simulink model "SimulinkFullblock"  (R2019b)
(part 5 of 5)

                                                                                                                                                                                                                                                                                                                                                                                                                                                                                                                                                                                                                                                                                                                                                                                                                                                                                                                                                                                                                                                                                                                                                                                                                                                                                                                                                                                                                                                                                                                                                                                                                                                                                                                                                                                                                                                      0,                                                                                                                                                                                                                                                                                                                                                                                                                                                                                                                                                                                                                                                                                                                                                                                                                                                                                                                                                                                                                                                                                                                                                                                                                                                                                                                                                                                                                                                                                                                                                                                                                                                                                                                                                                                                                                                                                                                                                                                                                                                                                                                                                                                                                                                                                                                                                                                                                                                                                                                                                                                                                                                                                                                                                                                                                                                                                                                                                                                                                                                                                                                                                                                                                                                                                                                                                                                                                                                                                                                                                                                                                                                                                                                                                                                                                                                                                                                                                                                                                                                                                                                                                                                                                                                                                                                                                                                                                                                                                                                                                                                                                                                                                                                                                                                                                                                                               -0.0175*sin(0.0175*q1 - 1.5708)*q1d,                                                                                                                                                         0,                                                                                                                                                                                                                                                                                                                                                                                                                                                                                                                                                                                                                                                                                                                                                                                                                                                                                                                                                                                                                                                                                                                                                                                                                                                                                                                                                                                                                                                                                                                                                                                                                                                                                                                                                                                                                                                                                                                                                                                                                                                                                                                                                                                                                                                                                                                                                                                                                                                                                                                                                                                                                                                                                                                                                                                                                                                                                                                                                                                                                                                                                                                                                                                                                                                                                                                                                                                                                                                                                                                                                                                                                                                                                                                                                                                                                                                                                                                                                                                                                                                                                                                                                                                                                                                                                                                                                                                                                                                                                                                                                                                                                                                                                                                                                                                                                                                                                                                                                                                                                                                                                                                                                                                                                                                                                                                                                                                                                                                                                                                                                                                                                                                                                                                                                                                                                                                                                                                                                                                                                                                                                                                                                                                                                                                                                                                                                                                                                                                                                                                                                                                                                                                                                                                                                                                                                                                                                                                                                                                                                                                                                                                                                                                                 0.0175*cos(0.0175*q1 - 1.5708)*sin(0.0175*q2 - 1.5708)*q1d + 0.0175*cos(0.0175*q2 - 1.5708)*sin(0.0175*q1 - 1.5708)*q2d,                                                                                                                                                                                                                                                                                                                                                                                                                                                                                                                                                                                                                                                                                                                                                                                                                                                                                                                                                                                                                                                                                                                                                                                                                                                                                                                                                                                                                                                                                                                                                                                                                                                                                                                                                                                                                                                                                                                                                                                                                                                                                                                                                                                                                                                                                                                                                                                                                                                                                                                                                                                                                                                                                                                                                                                                                                                                                                                                                                                                                                                                                                                                                                                                                                                                                                                                                                                                                                                                                                                                                                                                                                                                                                                                                                                                                                                                                                                                                                                                                                                                                                                                                                                                                                                                                                                                                                                                                                                                                                                                                                                                                                                                                                                                                                                                                                                                                                                                                                                                                                                                                                                                                                                                                                                                                                                                                                                                                                                                                                                                                                                                                                                                                                                                                                                                                                                                                                                                                                                                                                                                                                                                                                                                                                                                                                                                                                                                                                                                                                                                                                                                                                                                                                                                                                                                                                                                                                                                                                                                                                                                                                                                                                                                                                                                                      0.0175*cos(0.0175*q4 + 1.5708)*sin(0.0175*q1 - 1.5708)*q1d + 0.0175*cos(0.0175*q1 - 1.5708)*sin(0.0175*q4 + 1.5708)*q4d + 0.0175*cos(0.0175*q1 - 1.5708)*cos(0.0175*q2 - 1.5708)*sin(0.0175*q4 + 1.5708)*q1d + 0.0175*cos(0.0175*q2 - 1.5708)*cos(0.0175*q4 + 1.5708)*sin(0.0175*q1 - 1.5708)*q4d - 0.0175*sin(0.0175*q1 - 1.5708)*sin(0.0175*q2 - 1.5708)*sin(0.0175*q4 + 1.5708)*q2d,                                                                                                                                                                                                                                                                                                                                                                                                                                                                                                                                                                                                                                                                                                                                                                                                                                                                                                                                                                                                                                                                                                                                                                                                                                                                                                                                                                                                                                                                                                                                                                                                                                                                                                                                                                                                                                                                                                                                                                                                                                                                                                                                                                                                                                                                                                                                                                                                                                                                                                                                                                                                                                                                                                                                                                                                                                                                                                                                                                                                                                                                                                                                                                                                                                                                                                                                                                                                                                                                                                                                                                                                                                                                                                                                                                                                                                                                                                                                                                                                                                                                                                                                                                                                                                                                                                                                                                                                                                                                                                                                                                                                                                                                                                                                                                                                                                                                                                                                                                                                                                                                                                                                                                                                                                                                                                                                                                                                                                                                                                                                                                                                                                                                                                                                                                                                                                                                                                                                                                                                                                                                                                                                                                                                                                                                                                                                                                                                                                                                                                                                                                                                                                                                                                                                                                                                                                                                                                                                                                                                                                                                                                                                                                                                                                                                                                                                                                                                                                                                                                                                                                                                                                                                                                                                                                                                                                                                                                                                                                                                                                                                                                                                                                                                                                                                                                                                                                            0.0175*cos(0.0175*q5 + 1.5708)*q5d*(cos(0.0175*q1 - 1.5708)*sin(0.0175*q4 + 1.5708) + cos(0.0175*q2 - 1.5708)*cos(0.0175*q4 + 1.5708)*sin(0.0175*q1 - 1.5708)) - sin(0.0175*q5 + 1.5708)*(0.0175*sin(0.0175*q1 - 1.5708)*sin(0.0175*q4 + 1.5708)*q1d - 0.0175*cos(0.0175*q1 - 1.5708)*cos(0.0175*q4 + 1.5708)*q4d - 0.0175*cos(0.0175*q1 - 1.5708)*cos(0.0175*q2 - 1.5708)*cos(0.0175*q4 + 1.5708)*q1d + 0.0175*cos(0.0175*q4 + 1.5708)*sin(0.0175*q1 - 1.5708)*sin(0.0175*q2 - 1.5708)*q2d + 0.0175*cos(0.0175*q2 - 1.5708)*sin(0.0175*q1 - 1.5708)*sin(0.0175*q4 + 1.5708)*q4d) - 0.0175*cos(0.0175*q1 - 1.5708)*cos(0.0175*q5 + 1.5708)*sin(0.0175*q2 - 1.5708)*q1d - 0.0175*cos(0.0175*q2 - 1.5708)*cos(0.0175*q5 + 1.5708)*sin(0.0175*q1 - 1.5708)*q2d + 0.0175*sin(0.0175*q1 - 1.5708)*sin(0.0175*q2 - 1.5708)*sin(0.0175*q5 + 1.5708)*q5d;
                                                                                                                                                                                                                                                                                                                                                                                                                                                                                                                                                                                                                                                                                                                                                                                                                                                                                                                                                                                                                                                                                                                                                                                                                                                                                                                                                                                                                                                                                                                                                                                                                                                                                                                                                                                                                                                      0,                                                                                                                                                                                                                                                                                                                                                                                                                                                                                                                                                                                                                                                                                                                                                                                                                                                                                                                                                                                                                                                                                                                                                                                                                                                                                                                                                                                                                                                                                                                                                                                                                                                                                                                                                                                                                                                                                                                                                                                                                                                                                                                                                                                                                                                                                                                                                                                                                                                                                                                                                                                                                                                                                                                                                                                                                                                                                                                                                                                                                                                                                                                                                                                                                                                                                                                                                                                                                                                                                                                                                                                                                                                                                                                                                                                                                                                                                                                                                                                                                                                                                                                                                                                                                                                                                                                                                                                                                                                                                                                                                                                                                                                                                                                                                                                                                                                                                                                               0,                                                                                                                                                         0,                                                                                                                                                                                                                                                                                                                                                                                                                                                                                                                                                                                                                                                                                                                                                                                                                                                                                                                                                                                                                                                                                                                                                                                                                                                                                                                                                                                                                                                                                                                                                                                                                                                                                                                                                                                                                                                                                                                                                                                                                                                                                                                                                                                                                                                                                                                                                                                                                                                                                                                                                                                                                                                                                                                                                                                                                                                                                                                                                                                                                                                                                                                                                                                                                                                                                                                                                                                                                                                                                                                                                                                                                                                                                                                                                                                                                                                                                                                                                                                                                                                                                                                                                                                                                                                                                                                                                                                                                                                                                                                                                                                                                                                                                                                                                                                                                                                                                                                                                                                                                                                                                                                                                                                                                                                                                                                                                                                                                                                                                                                                                                                                                                                                                                                                                                                                                                                                                                                                                                                                                                                                                                                                                                                                                                                                                                                                                                                                                                                                                                                                                                                                                                                                                                                                                                                                                                                                                                                                                                                                                                                                                                                                                                                                                                                                                                         -0.0175*sin(0.0175*q2 - 1.5708)*q2d,                                                                                                                                                                                                                                                                                                                                                                                                                                                                                                                                                                                                                                                                                                                                                                                                                                                                                                                                                                                                                                                                                                                                                                                                                                                                                                                                                                                                                                                                                                                                                                                                                                                                                                                                                                                                                                                                                                                                                                                                                                                                                                                                                                                                                                                                                                                                                                                                                                                                                                                                                                                                                                                                                                                                                                                                                                                                                                                                                                                                                                                                                                                                                                                                                                                                                                                                                                                                                                                                                                                                                                                                                                                                                                                                                                                                                                                                                                                                                                                                                                                                                                                                                                                                                                                                                                                                                                                                                                                                                                                                                                                                                                                                                                                                                                                                                                                                                                                                                                                                                                                                                                                                                                                                                                                                                                                                                                                                                                                                                                                                                                                                                                                                                                                                                                                                                                                                                                                                                                                                                                                                                                                                                                                                                                                                                                                                                                                                                                                                                                                                                                                                                                                                                                                                                                                                                                                                                                                                                                                                                                                                                                                                                                                                                                                                                                                                                                                                                                                                                                                                                                                                               - 0.0175*cos(0.0175*q2 - 1.5708)*sin(0.0175*q4 + 1.5708)*q2d - 0.0175*cos(0.0175*q4 + 1.5708)*sin(0.0175*q2 - 1.5708)*q4d,                                                                                                                                                                                                                                                                                                                                                                                                                                                                                                                                                                                                                                                                                                                                                                                                                                                                                                                                                                                                                                                                                                                                                                                                                                                                                                                                                                                                                                                                                                                                                                                                                                                                                                                                                                                                                                                                                                                                                                                                                                                                                                                                                                                                                                                                                                                                                                                                                                                                                                                                                                                                                                                                                                                                                                                                                                                                                                                                                                                                                                                                                                                                                                                                                                                                                                                                                                                                                                                                                                                                                                                                                                                                                                                                                                                                                                                                                                                                                                                                                                                                                                                                                                                                                                                                                                                                                                                                                                                                                                                                                                                                                                                                                                                                                                                                                                                                                                                                                                                                                                                                                                                                                                                                                                                                                                                                                                                                                                                                                                                                                                                                                                                                                                                                                                                                                                                                                                                                                                                                                                                                                                                                                                                                                                                                                                                                                                                                                                                                                                                                                                                                                                                                                                                                                                                                                                                                                                                                                                                                                                                                                                                                                                                                                                                                                                                                                                                                                                                                                                                                                                                                                                                                                                                                                                                                                                                                                                                                                                                                                                                                                                                                                                                                                                                                                                                                                                                                                                                                                                                                                                                                                                                                                                                                                                                                                                                                                                                                  0.0175*cos(0.0175*q5 + 1.5708)*sin(0.0175*q2 - 1.5708)*q2d + 0.0175*cos(0.0175*q2 - 1.5708)*sin(0.0175*q5 + 1.5708)*q5d - 0.0175*cos(0.0175*q2 - 1.5708)*cos(0.0175*q4 + 1.5708)*sin(0.0175*q5 + 1.5708)*q2d - 0.0175*cos(0.0175*q4 + 1.5708)*cos(0.0175*q5 + 1.5708)*sin(0.0175*q2 - 1.5708)*q5d + 0.0175*sin(0.0175*q2 - 1.5708)*sin(0.0175*q4 + 1.5708)*sin(0.0175*q5 + 1.5708)*q4d];
                                                                                                                                                                                                                                                                                                                                                                                                                                                                                                                                                                                                                                                                                                                                                                                                                                                                                                                                                                                                                                                                                                                                                                                                                                                                                                                                                                                                                                                                                                                                                                                                                                                                                                                                                                                                                                                  
                                                                                                                                                                                                                                                                                                                                                                                                                                                                                                                                                                                                                                                                                                                                                                                                                                                                                                                                                                                                                                                                                                                                                                                                                                                                                                                                                                                                                                                                                                                                                                                                                                                                                                                             

J= [ - conj(L4)*(sin(0.0175*conj(q5) + 1.5708)*(cos(0.0175*conj(q1) - 1.5708)*sin(0.0175*conj(q4) + 1.5708) + cos(0.0175*conj(q2) - 1.5708)*cos(0.0175*conj(q4) + 1.5708)*sin(0.0175*conj(q1) - 1.5708)) - cos(0.0175*conj(q5) + 1.5708)*sin(0.0175*conj(q1) - 1.5708)*sin(0.0175*conj(q2) - 1.5708)) - sin(0.0175*conj(q1) - 1.5708)*sin(0.0175*conj(q2) - 1.5708)*(conj(q3) + conj(L2)) - sin(0.0175*conj(q1) - 1.5708)*sin(0.0175*conj(q2) - 1.5708)*conj(L3),                                                                                                                                                                                                                                                                                                                                                                                                                                                                                                                                                                                                                                                                                                                                                      cos(0.0175*conj(q1) - 1.5708)*(cos(0.0175*conj(q2) - 1.5708)*conj(L3) - conj(L4)*(cos(0.0175*conj(q2) - 1.5708)*cos(0.0175*conj(q5) + 1.5708) + cos(0.0175*conj(q4) + 1.5708)*sin(0.0175*conj(q2) - 1.5708)*sin(0.0175*conj(q5) + 1.5708)) + cos(0.0175*conj(q2) - 1.5708)*(conj(q3) + conj(L2))), cos(0.0175*q1 - 1.5708)*sin(0.0175*q2 - 1.5708),                                                                                                                                                                                                                                                                             sin(0.0175*conj(q1) - 1.5708)*sin(0.0175*conj(q2) - 1.5708)*(cos(0.0175*conj(q2) - 1.5708)*conj(L3) - conj(L4)*(cos(0.0175*conj(q2) - 1.5708)*cos(0.0175*conj(q5) + 1.5708) + cos(0.0175*conj(q4) + 1.5708)*sin(0.0175*conj(q2) - 1.5708)*sin(0.0175*conj(q5) + 1.5708)) + cos(0.0175*conj(q2) - 1.5708)*(conj(q3) + conj(L2)) - cos(0.0175*conj(q2) - 1.5708)*(conj(q3) + conj(L2))) - cos(0.0175*conj(q2) - 1.5708)*(conj(L4)*(sin(0.0175*conj(q5) + 1.5708)*(cos(0.0175*conj(q1) - 1.5708)*sin(0.0175*conj(q4) + 1.5708) + cos(0.0175*conj(q2) - 1.5708)*cos(0.0175*conj(q4) + 1.5708)*sin(0.0175*conj(q1) - 1.5708)) - cos(0.0175*conj(q5) + 1.5708)*sin(0.0175*conj(q1) - 1.5708)*sin(0.0175*conj(q2) - 1.5708)) + sin(0.0175*conj(q1) - 1.5708)*sin(0.0175*conj(q2) - 1.5708)*(conj(q3) + conj(L2)) - sin(0.0175*conj(q1) - 1.5708)*sin(0.0175*conj(q2) - 1.5708)*(conj(q3) + conj(L2)) + sin(0.0175*conj(q1) - 1.5708)*sin(0.0175*conj(q2) - 1.5708)*conj(L3)),                                                                                                                                                                                                                                                                                                                                                                                    (cos(0.0175*conj(q1) - 1.5708)*cos(0.0175*conj(q4) + 1.5708) - cos(0.0175*conj(q2) - 1.5708)*sin(0.0175*conj(q1) - 1.5708)*sin(0.0175*conj(q4) + 1.5708))*(cos(0.0175*conj(q2) - 1.5708)*conj(L3) - cos(0.0175*conj(q2) - 1.5708)*conj(L3) + conj(L4)*(cos(0.0175*conj(q2) - 1.5708)*cos(0.0175*conj(q5) + 1.5708) + cos(0.0175*conj(q4) + 1.5708)*sin(0.0175*conj(q2) - 1.5708)*sin(0.0175*conj(q5) + 1.5708)) - cos(0.0175*conj(q2) - 1.5708)*(conj(q3) + conj(L2)) + cos(0.0175*conj(q2) - 1.5708)*(conj(q3) + conj(L2))) + sin(0.0175*conj(q2) - 1.5708)*sin(0.0175*conj(q4) + 1.5708)*(conj(L4)*(sin(0.0175*conj(q5) + 1.5708)*(cos(0.0175*conj(q1) - 1.5708)*sin(0.0175*conj(q4) + 1.5708) + cos(0.0175*conj(q2) - 1.5708)*cos(0.0175*conj(q4) + 1.5708)*sin(0.0175*conj(q1) - 1.5708)) - cos(0.0175*conj(q5) + 1.5708)*sin(0.0175*conj(q1) - 1.5708)*sin(0.0175*conj(q2) - 1.5708)) + sin(0.0175*conj(q1) - 1.5708)*sin(0.0175*conj(q2) - 1.5708)*(conj(q3) + conj(L2)) - sin(0.0175*conj(q1) - 1.5708)*sin(0.0175*conj(q2) - 1.5708)*(conj(q3) + conj(L2)) + sin(0.0175*conj(q1) - 1.5708)*sin(0.0175*conj(q2) - 1.5708)*conj(L3) - sin(0.0175*conj(q1) - 1.5708)*sin(0.0175*conj(q2) - 1.5708)*conj(L3)),                                                                                                                                                                                                                                                                                                                                                                                                                     (cos(0.0175*conj(q2) - 1.5708)*cos(0.0175*conj(q5) + 1.5708) + cos(0.0175*conj(q4) + 1.5708)*sin(0.0175*conj(q2) - 1.5708)*sin(0.0175*conj(q5) + 1.5708))*(conj(L4)*(sin(0.0175*conj(q5) + 1.5708)*(cos(0.0175*conj(q1) - 1.5708)*sin(0.0175*conj(q4) + 1.5708) + cos(0.0175*conj(q2) - 1.5708)*cos(0.0175*conj(q4) + 1.5708)*sin(0.0175*conj(q1) - 1.5708)) - cos(0.0175*conj(q5) + 1.5708)*sin(0.0175*conj(q1) - 1.5708)*sin(0.0175*conj(q2) - 1.5708)) + sin(0.0175*conj(q1) - 1.5708)*sin(0.0175*conj(q2) - 1.5708)*(conj(q3) + conj(L2)) - sin(0.0175*conj(q1) - 1.5708)*sin(0.0175*conj(q2) - 1.5708)*(conj(q3) + conj(L2)) + sin(0.0175*conj(q1) - 1.5708)*sin(0.0175*conj(q2) - 1.5708)*conj(L3) - sin(0.0175*conj(q1) - 1.5708)*sin(0.0175*conj(q2) - 1.5708)*conj(L3)) - (sin(0.0175*conj(q5) + 1.5708)*(cos(0.0175*conj(q1) - 1.5708)*sin(0.0175*conj(q4) + 1.5708) + cos(0.0175*conj(q2) - 1.5708)*cos(0.0175*conj(q4) + 1.5708)*sin(0.0175*conj(q1) - 1.5708)) - cos(0.0175*conj(q5) + 1.5708)*sin(0.0175*conj(q1) - 1.5708)*sin(0.0175*conj(q2) - 1.5708))*(cos(0.0175*conj(q2) - 1.5708)*conj(L3) - cos(0.0175*conj(q2) - 1.5708)*conj(L3) + conj(L4)*(cos(0.0175*conj(q2) - 1.5708)*cos(0.0175*conj(q5) + 1.5708) + cos(0.0175*conj(q4) + 1.5708)*sin(0.0175*conj(q2) - 1.5708)*sin(0.0175*conj(q5) + 1.5708)) - cos(0.0175*conj(q2) - 1.5708)*(conj(q3) + conj(L2)) + cos(0.0175*conj(q2) - 1.5708)*(conj(q3) + conj(L2)));
   cos(0.0175*conj(q1) - 1.5708)*sin(0.0175*conj(q2) - 1.5708)*conj(L3) - conj(L4)*(sin(0.0175*conj(q5) + 1.5708)*(sin(0.0175*conj(q1) - 1.5708)*sin(0.0175*conj(q4) + 1.5708) - cos(0.0175*conj(q1) - 1.5708)*cos(0.0175*conj(q2) - 1.5708)*cos(0.0175*conj(q4) + 1.5708)) + cos(0.0175*conj(q1) - 1.5708)*cos(0.0175*conj(q5) + 1.5708)*sin(0.0175*conj(q2) - 1.5708)) + cos(0.0175*conj(q1) - 1.5708)*sin(0.0175*conj(q2) - 1.5708)*(conj(q3) + conj(L2)),                                                                                                                                                                                                                                                                                                                                                                                                                                                                                                                                                                                                                                                                                                                                                      sin(0.0175*conj(q1) - 1.5708)*(cos(0.0175*conj(q2) - 1.5708)*conj(L3) - conj(L4)*(cos(0.0175*conj(q2) - 1.5708)*cos(0.0175*conj(q5) + 1.5708) + cos(0.0175*conj(q4) + 1.5708)*sin(0.0175*conj(q2) - 1.5708)*sin(0.0175*conj(q5) + 1.5708)) + cos(0.0175*conj(q2) - 1.5708)*(conj(q3) + conj(L2))), sin(0.0175*q1 - 1.5708)*sin(0.0175*q2 - 1.5708),                                                                                                                                                                                                                                                                           - cos(0.0175*conj(q2) - 1.5708)*(conj(L4)*(sin(0.0175*conj(q5) + 1.5708)*(sin(0.0175*conj(q1) - 1.5708)*sin(0.0175*conj(q4) + 1.5708) - cos(0.0175*conj(q1) - 1.5708)*cos(0.0175*conj(q2) - 1.5708)*cos(0.0175*conj(q4) + 1.5708)) + cos(0.0175*conj(q1) - 1.5708)*cos(0.0175*conj(q5) + 1.5708)*sin(0.0175*conj(q2) - 1.5708)) - cos(0.0175*conj(q1) - 1.5708)*sin(0.0175*conj(q2) - 1.5708)*conj(L3) - cos(0.0175*conj(q1) - 1.5708)*sin(0.0175*conj(q2) - 1.5708)*(conj(q3) + conj(L2)) + cos(0.0175*conj(q1) - 1.5708)*sin(0.0175*conj(q2) - 1.5708)*(conj(q3) + conj(L2))) - cos(0.0175*conj(q1) - 1.5708)*sin(0.0175*conj(q2) - 1.5708)*(cos(0.0175*conj(q2) - 1.5708)*conj(L3) - conj(L4)*(cos(0.0175*conj(q2) - 1.5708)*cos(0.0175*conj(q5) + 1.5708) + cos(0.0175*conj(q4) + 1.5708)*sin(0.0175*conj(q2) - 1.5708)*sin(0.0175*conj(q5) + 1.5708)) + cos(0.0175*conj(q2) - 1.5708)*(conj(q3) + conj(L2)) - cos(0.0175*conj(q2) - 1.5708)*(conj(q3) + conj(L2))),                                                                                                                                                                                                                                                                                                                                                                                    (cos(0.0175*conj(q4) + 1.5708)*sin(0.0175*conj(q1) - 1.5708) + cos(0.0175*conj(q1) - 1.5708)*cos(0.0175*conj(q2) - 1.5708)*sin(0.0175*conj(q4) + 1.5708))*(cos(0.0175*conj(q2) - 1.5708)*conj(L3) - cos(0.0175*conj(q2) - 1.5708)*conj(L3) + conj(L4)*(cos(0.0175*conj(q2) - 1.5708)*cos(0.0175*conj(q5) + 1.5708) + cos(0.0175*conj(q4) + 1.5708)*sin(0.0175*conj(q2) - 1.5708)*sin(0.0175*conj(q5) + 1.5708)) - cos(0.0175*conj(q2) - 1.5708)*(conj(q3) + conj(L2)) + cos(0.0175*conj(q2) - 1.5708)*(conj(q3) + conj(L2))) + sin(0.0175*conj(q2) - 1.5708)*sin(0.0175*conj(q4) + 1.5708)*(conj(L4)*(sin(0.0175*conj(q5) + 1.5708)*(sin(0.0175*conj(q1) - 1.5708)*sin(0.0175*conj(q4) + 1.5708) - cos(0.0175*conj(q1) - 1.5708)*cos(0.0175*conj(q2) - 1.5708)*cos(0.0175*conj(q4) + 1.5708)) + cos(0.0175*conj(q1) - 1.5708)*cos(0.0175*conj(q5) + 1.5708)*sin(0.0175*conj(q2) - 1.5708)) - cos(0.0175*conj(q1) - 1.5708)*sin(0.0175*conj(q2) - 1.5708)*conj(L3) + cos(0.0175*conj(q1) - 1.5708)*sin(0.0175*conj(q2) - 1.5708)*conj(L3) - cos(0.0175*conj(q1) - 1.5708)*sin(0.0175*conj(q2) - 1.5708)*(conj(q3) + conj(L2)) + cos(0.0175*conj(q1) - 1.5708)*sin(0.0175*conj(q2) - 1.5708)*(conj(q3) + conj(L2))),                                                                                                                                                                                                                                                                                                                                                                                                                     (cos(0.0175*conj(q2) - 1.5708)*cos(0.0175*conj(q5) + 1.5708) + cos(0.0175*conj(q4) + 1.5708)*sin(0.0175*conj(q2) - 1.5708)*sin(0.0175*conj(q5) + 1.5708))*(conj(L4)*(sin(0.0175*conj(q5) + 1.5708)*(sin(0.0175*conj(q1) - 1.5708)*sin(0.0175*conj(q4) + 1.5708) - cos(0.0175*conj(q1) - 1.5708)*cos(0.0175*conj(q2) - 1.5708)*cos(0.0175*conj(q4) + 1.5708)) + cos(0.0175*conj(q1) - 1.5708)*cos(0.0175*conj(q5) + 1.5708)*sin(0.0175*conj(q2) - 1.5708)) - cos(0.0175*conj(q1) - 1.5708)*sin(0.0175*conj(q2) - 1.5708)*conj(L3) + cos(0.0175*conj(q1) - 1.5708)*sin(0.0175*conj(q2) - 1.5708)*conj(L3) - cos(0.0175*conj(q1) - 1.5708)*sin(0.0175*conj(q2) - 1.5708)*(conj(q3) + conj(L2)) + cos(0.0175*conj(q1) - 1.5708)*sin(0.0175*conj(q2) - 1.5708)*(conj(q3) + conj(L2))) - (sin(0.0175*conj(q5) + 1.5708)*(sin(0.0175*conj(q1) - 1.5708)*sin(0.0175*conj(q4) + 1.5708) - cos(0.0175*conj(q1) - 1.5708)*cos(0.0175*conj(q2) - 1.5708)*cos(0.0175*conj(q4) + 1.5708)) + cos(0.0175*conj(q1) - 1.5708)*cos(0.0175*conj(q5) + 1.5708)*sin(0.0175*conj(q2) - 1.5708))*(cos(0.0175*conj(q2) - 1.5708)*conj(L3) - cos(0.0175*conj(q2) - 1.5708)*conj(L3) + conj(L4)*(cos(0.0175*conj(q2) - 1.5708)*cos(0.0175*conj(q5) + 1.5708) + cos(0.0175*conj(q4) + 1.5708)*sin(0.0175*conj(q2) - 1.5708)*sin(0.0175*conj(q5) + 1.5708)) - cos(0.0175*conj(q2) - 1.5708)*(conj(q3) + conj(L2)) + cos(0.0175*conj(q2) - 1.5708)*(conj(q3) + conj(L2)));
                                                                                                                                                                                                                                                                                                                                                                                                                                                                                                     0, - cos(0.0175*conj(q1) - 1.5708)*(cos(0.0175*conj(q1) - 1.5708)*sin(0.0175*conj(q2) - 1.5708)*conj(L3) - conj(L4)*(sin(0.0175*conj(q5) + 1.5708)*(sin(0.0175*conj(q1) - 1.5708)*sin(0.0175*conj(q4) + 1.5708) - cos(0.0175*conj(q1) - 1.5708)*cos(0.0175*conj(q2) - 1.5708)*cos(0.0175*conj(q4) + 1.5708)) + cos(0.0175*conj(q1) - 1.5708)*cos(0.0175*conj(q5) + 1.5708)*sin(0.0175*conj(q2) - 1.5708)) + cos(0.0175*conj(q1) - 1.5708)*sin(0.0175*conj(q2) - 1.5708)*(conj(q3) + conj(L2))) - sin(0.0175*conj(q1) - 1.5708)*(conj(L4)*(sin(0.0175*conj(q5) + 1.5708)*(cos(0.0175*conj(q1) - 1.5708)*sin(0.0175*conj(q4) + 1.5708) + cos(0.0175*conj(q2) - 1.5708)*cos(0.0175*conj(q4) + 1.5708)*sin(0.0175*conj(q1) - 1.5708)) - cos(0.0175*conj(q5) + 1.5708)*sin(0.0175*conj(q1) - 1.5708)*sin(0.0175*conj(q2) - 1.5708)) + sin(0.0175*conj(q1) - 1.5708)*sin(0.0175*conj(q2) - 1.5708)*(conj(q3) + conj(L2)) + sin(0.0175*conj(q1) - 1.5708)*sin(0.0175*conj(q2) - 1.5708)*conj(L3)),                            cos(0.0175*q2 - 1.5708), sin(0.0175*conj(q1) - 1.5708)*sin(0.0175*conj(q2) - 1.5708)*(conj(L4)*(sin(0.0175*conj(q5) + 1.5708)*(sin(0.0175*conj(q1) - 1.5708)*sin(0.0175*conj(q4) + 1.5708) - cos(0.0175*conj(q1) - 1.5708)*cos(0.0175*conj(q2) - 1.5708)*cos(0.0175*conj(q4) + 1.5708)) + cos(0.0175*conj(q1) - 1.5708)*cos(0.0175*conj(q5) + 1.5708)*sin(0.0175*conj(q2) - 1.5708)) - cos(0.0175*conj(q1) - 1.5708)*sin(0.0175*conj(q2) - 1.5708)*conj(L3) - cos(0.0175*conj(q1) - 1.5708)*sin(0.0175*conj(q2) - 1.5708)*(conj(q3) + conj(L2)) + cos(0.0175*conj(q1) - 1.5708)*sin(0.0175*conj(q2) - 1.5708)*(conj(q3) + conj(L2))) + cos(0.0175*conj(q1) - 1.5708)*sin(0.0175*conj(q2) - 1.5708)*(conj(L4)*(sin(0.0175*conj(q5) + 1.5708)*(cos(0.0175*conj(q1) - 1.5708)*sin(0.0175*conj(q4) + 1.5708) + cos(0.0175*conj(q2) - 1.5708)*cos(0.0175*conj(q4) + 1.5708)*sin(0.0175*conj(q1) - 1.5708)) - cos(0.0175*conj(q5) + 1.5708)*sin(0.0175*conj(q1) - 1.5708)*sin(0.0175*conj(q2) - 1.5708)) + sin(0.0175*conj(q1) - 1.5708)*sin(0.0175*conj(q2) - 1.5708)*(conj(q3) + conj(L2)) - sin(0.0175*conj(q1) - 1.5708)*sin(0.0175*conj(q2) - 1.5708)*(conj(q3) + conj(L2)) + sin(0.0175*conj(q1) - 1.5708)*sin(0.0175*conj(q2) - 1.5708)*conj(L3)), (cos(0.0175*conj(q4) + 1.5708)*sin(0.0175*conj(q1) - 1.5708) + cos(0.0175*conj(q1) - 1.5708)*cos(0.0175*conj(q2) - 1.5708)*sin(0.0175*conj(q4) + 1.5708))*(conj(L4)*(sin(0.0175*conj(q5) + 1.5708)*(cos(0.0175*conj(q1) - 1.5708)*sin(0.0175*conj(q4) + 1.5708) + cos(0.0175*conj(q2) - 1.5708)*cos(0.0175*conj(q4) + 1.5708)*sin(0.0175*conj(q1) - 1.5708)) - cos(0.0175*conj(q5) + 1.5708)*sin(0.0175*conj(q1) - 1.5708)*sin(0.0175*conj(q2) - 1.5708)) + sin(0.0175*conj(q1) - 1.5708)*sin(0.0175*conj(q2) - 1.5708)*(conj(q3) + conj(L2)) - sin(0.0175*conj(q1) - 1.5708)*sin(0.0175*conj(q2) - 1.5708)*(conj(q3) + conj(L2)) + sin(0.0175*conj(q1) - 1.5708)*sin(0.0175*conj(q2) - 1.5708)*conj(L3) - sin(0.0175*conj(q1) - 1.5708)*sin(0.0175*conj(q2) - 1.5708)*conj(L3)) - (cos(0.0175*conj(q1) - 1.5708)*cos(0.0175*conj(q4) + 1.5708) - cos(0.0175*conj(q2) - 1.5708)*sin(0.0175*conj(q1) - 1.5708)*sin(0.0175*conj(q4) + 1.5708))*(conj(L4)*(sin(0.0175*conj(q5) + 1.5708)*(sin(0.0175*conj(q1) - 1.5708)*sin(0.0175*conj(q4) + 1.5708) - cos(0.0175*conj(q1) - 1.5708)*cos(0.0175*conj(q2) - 1.5708)*cos(0.0175*conj(q4) + 1.5708)) + cos(0.0175*conj(q1) - 1.5708)*cos(0.0175*conj(q5) + 1.5708)*sin(0.0175*conj(q2) - 1.5708)) - cos(0.0175*conj(q1) - 1.5708)*sin(0.0175*conj(q2) - 1.5708)*conj(L3) + cos(0.0175*conj(q1) - 1.5708)*sin(0.0175*conj(q2) - 1.5708)*conj(L3) - cos(0.0175*conj(q1) - 1.5708)*sin(0.0175*conj(q2) - 1.5708)*(conj(q3) + conj(L2)) + cos(0.0175*conj(q1) - 1.5708)*sin(0.0175*conj(q2) - 1.5708)*(conj(q3) + conj(L2))), (sin(0.0175*conj(q5) + 1.5708)*(cos(0.0175*conj(q1) - 1.5708)*sin(0.0175*conj(q4) + 1.5708) + cos(0.0175*conj(q2) - 1.5708)*cos(0.0175*conj(q4) + 1.5708)*sin(0.0175*conj(q1) - 1.5708)) - cos(0.0175*conj(q5) + 1.5708)*sin(0.0175*conj(q1) - 1.5708)*sin(0.0175*conj(q2) - 1.5708))*(conj(L4)*(sin(0.0175*conj(q5) + 1.5708)*(sin(0.0175*conj(q1) - 1.5708)*sin(0.0175*conj(q4) + 1.5708) - cos(0.0175*conj(q1) - 1.5708)*cos(0.0175*conj(q2) - 1.5708)*cos(0.0175*conj(q4) + 1.5708)) + cos(0.0175*conj(q1) - 1.5708)*cos(0.0175*conj(q5) + 1.5708)*sin(0.0175*conj(q2) - 1.5708)) - cos(0.0175*conj(q1) - 1.5708)*sin(0.0175*conj(q2) - 1.5708)*conj(L3) + cos(0.0175*conj(q1) - 1.5708)*sin(0.0175*conj(q2) - 1.5708)*conj(L3) - cos(0.0175*conj(q1) - 1.5708)*sin(0.0175*conj(q2) - 1.5708)*(conj(q3) + conj(L2)) + cos(0.0175*conj(q1) - 1.5708)*sin(0.0175*conj(q2) - 1.5708)*(conj(q3) + conj(L2))) - (sin(0.0175*conj(q5) + 1.5708)*(sin(0.0175*conj(q1) - 1.5708)*sin(0.0175*conj(q4) + 1.5708) - cos(0.0175*conj(q1) - 1.5708)*cos(0.0175*conj(q2) - 1.5708)*cos(0.0175*conj(q4) + 1.5708)) + cos(0.0175*conj(q1) - 1.5708)*cos(0.0175*conj(q5) + 1.5708)*sin(0.0175*conj(q2) - 1.5708))*(conj(L4)*(sin(0.0175*conj(q5) + 1.5708)*(cos(0.0175*conj(q1) - 1.5708)*sin(0.0175*conj(q4) + 1.5708) + cos(0.0175*conj(q2) - 1.5708)*cos(0.0175*conj(q4) + 1.5708)*sin(0.0175*conj(q1) - 1.5708)) - cos(0.0175*conj(q5) + 1.5708)*sin(0.0175*conj(q1) - 1.5708)*sin(0.0175*conj(q2) - 1.5708)) + sin(0.0175*conj(q1) - 1.5708)*sin(0.0175*conj(q2) - 1.5708)*(conj(q3) + conj(L2)) - sin(0.0175*conj(q1) - 1.5708)*sin(0.0175*conj(q2) - 1.5708)*(conj(q3) + conj(L2)) + sin(0.0175*conj(q1) - 1.5708)*sin(0.0175*conj(q2) - 1.5708)*conj(L3) - sin(0.0175*conj(q1) - 1.5708)*sin(0.0175*conj(q2) - 1.5708)*conj(L3));
                                                                                                                                                                                                                                                                                                                                                                                                                                                                                                     0,                                                                                                                                                                                                                                                                                                                                                                                                                                                                                                                                                                                                                                                                                                                                                                                                                                                                                                                                                                                                                                                       -sin(0.0175*q1 - 1.5708),                                                     0,                                                                                                                                                                                                                                                                                                                                                                                                                                                                                                                                                                                                                                                                                                                                                                                                                                                                                                                                                                                                                                                                                                                                                                                                                                                                                       cos(0.0175*q1 - 1.5708)*sin(0.0175*q2 - 1.5708),                                                                                                                                                                                                                                                                                                                                                                                                                                                                                                                                                                                                                                                                                                                                                                                                                                                                                                                                                                                                                                                                                                                                                                                                                                                                                                                                                                                                                                                                                                                                                                            cos(0.0175*q4 + 1.5708)*sin(0.0175*q1 - 1.5708) + cos(0.0175*q1 - 1.5708)*cos(0.0175*q2 - 1.5708)*sin(0.0175*q4 + 1.5708),                                                                                                                                                                                                                                                                                                                                                                                                                                                                                                                                                                                                                                                                                                                                                                                                                                                                                                                                                                                                                                                                                                                                                                                                                                                                                                                                                                                                                                                                                                                                                                                                                                                                                                                                          - sin(0.0175*q5 + 1.5708)*(sin(0.0175*q1 - 1.5708)*sin(0.0175*q4 + 1.5708) - cos(0.0175*q1 - 1.5708)*cos(0.0175*q2 - 1.5708)*cos(0.0175*q4 + 1.5708)) - cos(0.0175*q1 - 1.5708)*cos(0.0175*q5 + 1.5708)*sin(0.0175*q2 - 1.5708);
                                                                                                                                                                                                                                                                                                                                                                                                                                                                                                     0,                                                                                                                                                                                                                                                                                                                                                                                                                                                                                                                                                                                                                                                                                                                                                                                                                                                                                                                                                                                                                                                        cos(0.0175*q1 - 1.5708),                                                     0,                                                                                                                                                                                                                                                                                                                                                                                                                                                                                                                                                                                                                                                                                                                                                                                                                                                                                                                                                                                                                                                                                                                                                                                                                                                                                       sin(0.0175*q1 - 1.5708)*sin(0.0175*q2 - 1.5708),                                                                                                                                                                                                                                                                                                                                                                                                                                                                                                                                                                                                                                                                                                                                                                                                                                                                                                                                                                                                                                                                                                                                                                                                                                                                                                                                                                                                                                                                                                                                                                            cos(0.0175*q2 - 1.5708)*sin(0.0175*q1 - 1.5708)*sin(0.0175*q4 + 1.5708) - cos(0.0175*q1 - 1.5708)*cos(0.0175*q4 + 1.5708),                                                                                                                                                                                                                                                                                                                                                                                                                                                                                                                                                                                                                                                                                                                                                                                                                                                                                                                                                                                                                                                                                                                                                                                                                                                                                                                                                                                                                                                                                                                                                                                                                                                                                                                                            sin(0.0175*q5 + 1.5708)*(cos(0.0175*q1 - 1.5708)*sin(0.0175*q4 + 1.5708) + cos(0.0175*q2 - 1.5708)*cos(0.0175*q4 + 1.5708)*sin(0.0175*q1 - 1.5708)) - cos(0.0175*q5 + 1.5708)*sin(0.0175*q1 - 1.5708)*sin(0.0175*q2 - 1.5708);
                                                                                                                                                                                                                                                                                                                                                                                                                                                                                                     1,                                                                                                                                                                                                                                                                                                                                                                                                                                                                                                                                                                                                                                                                                                                                                                                                                                                                                                                                                                                                                                                                                 0,                                                     0,                                                                                                                                                                                                                                                                                                                                                                                                                                                                                                                                                                                                                                                                                                                                                                                                                                                                                                                                                                                                                                                                                                                                                                                                                                                                                                                  cos(0.0175*q2 - 1.5708),                                                                                                                                                                                                                                                                                                                                                                                                                                                                                                                                                                                                                                                                                                                                                                                                                                                                                                                                                                                                                                                                                                                                                                                                                                                                                                                                                                                                                                                                                                                                                                                                                                                              -sin(0.0175*q2 - 1.5708)*sin(0.0175*q4 + 1.5708),                                                                                                                                                                                                                                                                                                                                                                                                                                                                                                                                                                                                                                                                                                                                                                                                                                                                                                                                                                                                                                                                                                                                                                                                                                                                                                                                                                                                                                                                                                                                                                                                                                                                                                                                                                                                                                                          - cos(0.0175*q2 - 1.5708)*cos(0.0175*q5 + 1.5708) - cos(0.0175*q4 + 1.5708)*sin(0.0175*q2 - 1.5708)*sin(0.0175*q5 + 1.5708)];
 


qdd= inv(J) * ([xdd;ydd;zdd;wxdd;wydd;wzdd]-Jdev*[q1d;q2d;q3d;q4d;q5d;q6d]);
